simulink model "q2section5"  (R2020a)
settings: Solver=VariableStepAuto  StartTime=0.0  StopTime=12  RelTol=1e-3
values from neighbouring files (symbols this model uses):
  A = 5*10^(-3)    (= 0.005)    [q2.m]
  beta = 10^9    (= 1000000000)    [q2.m]
  cf = 9*10^3    (= 9000)    [q2.m]
  ct = 2*10^(-10)    (= 2e-10)    [q2.m]
  dens = 850    [q2.m]
  g = 9.81    [q2.m]
  Kq = 2*10^(-3)    (= 0.002)    [q2.m]
  m = 100    [q2.m]
  mL = 1000    [q2.m]
  Ps = 7*10^6    (= 7000000)    [q2.m]
  V = 11*10^(-3)    (= 0.011)    [q2.m]
  xv_eq = (ct*m*g)/(A*Kq*sqrt((Ps-(m*g/A))/dens))    [q2.m]
libraries: cstblocks x2, simulink x1
settings Model: Creator=Nir Lalum  LastModifiedBy=Nir Lalum
settings SFSimCC: CustomCodeUndefinedFunction=UseInterfaceOnly

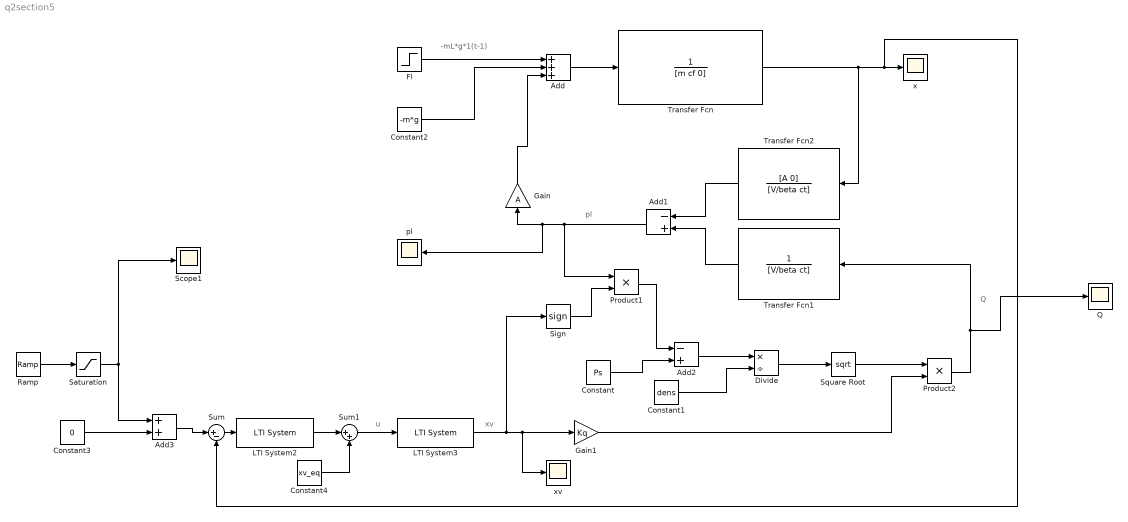
== system q2section5 ==
  note: -mL*g*1(t-1)
  note: pl
  note: xv
  note: Q
  note: u
  Add : Sum  Inputs=+++
  Add1 : Sum  Inputs=-+
  Add2 : Sum  Inputs=-+
  Add3 : Sum
  Constant : Constant  Value=Ps
  Constant1 : Constant  Value=dens
  Constant2 : Constant  Value=-m*g
  Constant3 : Constant  Value=0
  Constant4 : Constant  Value=xv_eq
  Divide : Product  Inputs=*/
  Fl : Step  Time=0  After=-mL*g  SampleTime=0
  Gain : Gain  Gain=A
  Gain1 : Gain  Gain=Kq
  LTI System2 : cstblocks/LTI System  sys=Ctot  IC=[]
  LTI System3 : cstblocks/LTI System  sys=Pvalve  IC=[]
  Product1 : Product
  Product2 : Product
  Q : Scope
  Ramp : simulink/Sources/Ramp  slope=0.18  start=1  InitialOutput=0
  Saturation : Saturate  UpperLimit=1
  Scope1 : Scope
  Sign : Signum
  Square Root : Sqrt  SaturateOnIntegerOverflow=on
  Sum : Sum  Inputs=|+-
  Sum1 : Sum  Inputs=|++
  Transfer Fcn : TransferFcn  Denominator=[m cf 0]
  Transfer Fcn1 : TransferFcn  Denominator=[V/beta ct]
  Transfer Fcn2 : TransferFcn  Numerator=[A 0]  Denominator=[V/beta ct]
  pl : Scope
  x : Scope
  "xv " : Scope
  wires:
  Add1/1 -> Product1/1, pl/1, Gain/1
  Square Root/1 -> Product2/1
  Gain/1 -> Add/3
  Constant1/1 -> Divide/2
  Gain1/1 -> Product2/2
  Divide/1 -> Square Root/1
  Constant2/1 -> Add/2
  Product1/1 -> Add2/1
  Add/1 -> Transfer Fcn/1
  Transfer Fcn2/1 -> Add1/1
  Fl/1 -> Add/1
  Constant/1 -> Add2/2
  Add2/1 -> Divide/1
  Product2/1 -> Q/1, Transfer Fcn1/1
  Sign/1 -> Product1/2
  Transfer Fcn1/1 -> Add1/2
  Sum/1 -> LTI System2/1
  Transfer Fcn/1 -> Transfer Fcn2/1, Sum/2, x/1
  LTI System3/1 -> "xv "/1, Gain1/1, Sign/1
  Constant3/1 -> Add3/2
  Add3/1 -> Sum/1
  Ramp/1 -> Saturation/1
  Saturation/1 -> Add3/1, Scope1/1
  LTI System2/1 -> Sum1/1
  Sum1/1 -> LTI System3/1
  Constant4/1 -> Sum1/2
